simulink model "Furuta_Model"  (R2015a)
settings: Solver=ode3  SolverMode=SingleTasking  StartTime=0.0  StopTime=Inf  FixedStep=0.0001  RelTol=1e-3
PostLoadFcn:
  | , if any(exist('dsrtsu_mdlpostloadfcn', 'file') == [2, 3, 6]), try dsrtsu_mdlpostloadfcn('Execute', bdroot); catch fprintf('Error in PostLoadFcn (dsrtsu_mdlpostloadfcn) for model "%s":\n %s\n', bdroot, lasterr); end, end,
values from neighbouring files (symbols this model uses):
  alpha = J + (M+m1/3+m2)*L1^2    (= 0.002160093571)    [Furuta_Constants.m]
  beta = (M + m2/3)*L2^2    (= 0.00192796261667)    [Furuta_Constants.m]
  gamma = (M + m2/2)*L2*L1    (= 0.0009263333625)    [Furuta_Constants.m]
  initial_state = pi    (= 3.14159265359)    [Furuta_Constants.m]
  kb = 6e-4    (= 0.0006)    [Furuta_Constants.m]
  ke = 0.182    [Furuta_Constants.m]
  Re = 3.6    [Furuta_Constants.m]
  sigma = (M + m2/2)*g*L2    (= 0.0951054975)    [Furuta_Constants.m]
libraries: rti2202miolib x8, simulink_extras x1
settings Model: DSRTSU_INTERNAL_RTI_VER=450  DSRTSU_INTERNAL_RTI_TYPE=rti1006  DSRTSU_INTERNAL_RTIFPGA=40  CovMetricSettings=dwe  CovHtmlReporting=off  covSaveCumulativeToWorkspaceVar=off  CovSaveSingleToWorkspaceVar=off  CovExternalEMLEnable=on  Creator=Marcelo  LastModifiedBy=NSEE
settings SolverCC: ZeroCrossControl=DisableAll
settings DataIOCC: LimitDataPoints=off  SaveFormat=Dataset
settings OptimizationCC: BlockReduction=off  OptimizeBlockIOStorage=off  BufferReuse=off  GlobalBufferReuse=off  ExpressionFolding=off  LocalBlockOutputs=off
settings DebuggingCC: ParameterOverflowMsg=warning  SFUnexpectedBacktrackingDiag=error  SFNoUnconditionalDefaultTransitionDiag=error
settings HardwareCC: ProdBitPerPointer=64  ProdLargestAtomicFloat=Float  ProdIntDivRoundTo=Zero  ProdEndianess=LittleEndian  ProdHWDeviceType=Generic->Custom  TargetIntDivRoundTo=Zero  TargetEndianess=LittleEndian  TargetHWDeviceType=Generic->Custom
settings ModelReferenceCC: ModelReferenceMinAlgLoopOccurrences=on  PropagateSignalLabelsOutOfModel=on
settings RTWCC: SystemTargetFile=rti1006.tlc  MakeCommand=make_rti  TemplateMakefile=rti1006.tmf  Description=dSPACE DS1006 Hardware Platform
settings STFCustomTargetCC: GenerateSampleERTMain=off  ParMdlRefBuildCompliant=on  GeneratePreprocessorConditionals=Disable all  ERTCustomFileBanners=off  SupportNonInlinedSFcns=on  SupportVariableSizeSignals=off  MATLABClassNameForMDSCustomization=Simulink.SoftwareTarget.GRTCustomization  GRTInterface=on  SystemTargetFile=rti1006.tlc
settings GRTTargetCC: CompOptLevelCompliant=off  ConcurrentExecutionCompliant=off  CombineOutputUpdateFcns=off  MatFileLogging=off  CPPClassGenCompliant=off  GRTInterface=on  ExtModeMexFile=noextcomm

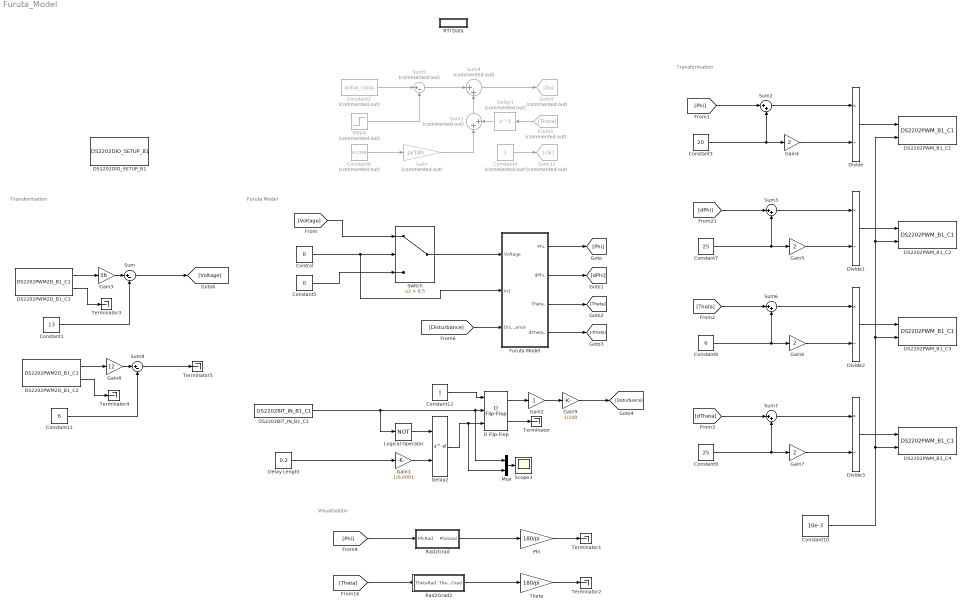
== system Furuta_Model ==
  note: Transformation
  note: Transformation
  note: Furuta Model
  note: Visualisation
  Constant1 : Constant  Value=13
  Constant10 : Constant  Value=10e-3
  Constant11 : Constant  Value=6
  Constant12 : Constant  OutDataTypeStr=boolean
  Constant2 : Constant  Commented=on  Value=initial_state
  Constant3 : Constant  Value=20
  Constant4 : Constant  Commented=on
  Constant5 : Constant  Value=0
  Constant6 : Constant  Commented=on  Value=9.2399
  Constant7 : Constant  Value=25
  Constant8 : Constant  Value=6
  Constant9 : Constant  Value=25
  Control : Constant  Value=0
  D Flip-Flop : simulink_extras/Flip Flops/D Flip-Flop
  DS2202BIT_IN_B1_C1 : rti2202miolib/DS2202BIT_IN_B1_C1  Reserved1=[]  Reserved2=[]  Reserved3=[]  Reserved4=[]  DSProperties=struct('RTI',struct('Version',uint32(1),'BlockType',struct('isSLSource',uint8(1),'isSLSink',uint8(0),'isHWSource',uint8(1),'isHWSink',uint8(0),'isSetup',uint8(0),'isInline',uint8(1),'isNonInline',uint8(0),'isInterrupt',uint8(0),'isChannelwise',uint8(1)),'IOBoardType',{{'DS2202','MIO'}},'UnitType','BIT','Identifier','BITINCH','DialogType','ML','BlockSet','NONE','SlaveProcessor','NONE'))  RTIBlockInterface=struct('OutputPortsWidth',int32(1),'OutputPortsDataType',{{'SS_BOOLEAN'}},'OutputPortsActive',1,'OutputPortsName',{{'BITCH_out'}},'BlockDisplay',{{['BIT IN\n Channelwise'],'center'}},'IconTransparency','off','InitLevel',2,'DialogFcn','gui2202bitinch','BlockName',struct('Token',{{'DS2202BIT_IN_B','_C'}},'BlockParam',{{'BoardNo','ChannelNo'}}),'MaskDescription',['Provides channelwise read access to the digital input.'])  RTIBlockParameters=struct('BoardNo',{{1,'ON',[1 16]}},'ChannelNo',{{1,'ON',[1 38]}},'TLCFileName',{{'rti2202inch','OFF',[]}})  RTISFcnParameters=struct('BoardNo','int32','ChannelNo','int32','TLCFileName','char')  RTIBlockParaDefault=struct('BoardNo',1,'ChannelNo',1,'TLCFileName','rti2202inch')
  DS2202DIO_SETUP_B1 : rti2202miolib/DS2202DIO_SETUP_B1  Reserved1=[]  Reserved2=[]  Reserved3=[]  Reserved4=[]  DSProperties=struct('RTI',struct('Version',uint32(2),'BlockType',struct('isSLSource',uint8(0),'isSLSink',uint8(0),'isHWSource',uint8(0),'isHWSink',uint8(0),'isSetup',uint8(1),'isInline',uint8(1),'isNonInline',uint8(0),'isInterrupt',uint8(0),'isChannelwise',uint8(0)),'IOBoardType',{{'DS2202','MIO'}},'UnitType','SETUP','Identifier','SETUP','DialogType','ML','BlockSet','NONE','SlaveProcessor','NONE'))  RTIBlockInterface=struct('OutputPortsWidth',int32(0),'OutputPortsActive',0,'BlockDisplay',{{['Digital I/O\n SETUP'],'center'}},'IconTransparency','on','InitLevel',2,'DialogFcn','gui2202diosetup','BlockName',struct('Token',{{'DS2202DIO_SETUP_B'}},'BlockParam',{{'BoardNo'}}),'MaskDescription',['Configures the threshold level and the termination mode for all digital IO'])  RTIBlockParameters=struct('BoardNo',{{1,'ON',[1 16]}},'TermMode',{{0,'OFF',[0 1]}},'BitInThresholdLevelCh1',{{'2.5','OFF',[1 23.8]}},'BitInThresholdLevelCh2',{{'2.5','OFF',[1 23.8]}},'BitInThresholdLevelCh3',{{'2.5','OFF',[1 23.8]}},'BitInThresholdLevelCh4',{{'2.5','OFF',[1 23.8]}},'BitInThresholdLevelCh5',{{'2.5','OFF',[1 23.8]}},'BitInThresholdLevelCh6',{{'2.5','OFF',[1 23.8]}},'BitInThresholdLevelCh7',{{'2.5','OFF',[1 23.8]}},'BitInThresholdLevelCh8',{{'2.5','OFF',[1 23.8]}},'BitInThresholdLevelCh9',{{'2.5','OFF',[1 23.8]}},'BitInThresholdLevelCh10',{{'2.5','OFF',[1 23.8]}},'BitInThresholdLevelCh11',{{'2.5','OFF',[1 23.8]}},'BitInThresholdLevelCh12',{{'2.5','OFF',[1 23.8]}},'BitInThresholdLevelCh13',{{'2.5','OFF',[1 23.8]}},'BitInThresholdLevelCh14',{{'2.5','OFF',[1 23.8]}},'BitInThresholdLevelCh15',{{'2.5','OFF',[1 23.8]}},'BitInThresholdLevelCh16',{{'2.5','OFF',[1 23.8]}},'BitInThresholdLevelCh17',{{'2.5','OFF',[1 23.8]}},'BitInThresholdLevelCh18',{{'2.5','OFF',[1 23.8]}},'BitInThresholdLevelCh19',{{'2.5','OFF',[1 23.8]}},'BitInThresholdLevelCh20',{{'2.5','OFF',[1 23.8]}},'BitInThresholdLevelCh21',{{'2.5','OFF',[1 23.8]}},'BitInThresholdLevelCh22',{{'2.5','OFF',[1 23.8]}},'BitInThresholdLevelCh23',{{'2.5','OFF',[1 23.8]}},'BitInThresholdLevelCh24',{{'2.5','OFF',[1 23.8]}},'BitInThresholdLevelCh25',{{'2.5','OFF',[1 23.8]}},'BitInThresholdLevelCh25_32',{{'2.5','OFF',[1 23.8]}},'BitInThresholdLevelCh33_38',{{'2.5','OFF',[1 23.8]}},'BitOutVBATRailsLOW',{{[1 1 1 1 1 1 1 1 1 1 1 1 1 1 1 1 1],'OFF',[]}},'BitOutVBATRailsVBAT1',{{[1 1 1 1 1 1 1 1 1 1 1 1 1 1 1 1 1],'OFF',[]}},'BitOutVBATRailsVBAT2',{{[0 0 0 0 0 0 0 0 0 0 0 0 0 0 0 0 0],'OFF',[]}},'PWMOutVBATRailsLOW',{{[1 1 1 1 1 1 1 1 1 1],'OFF',[]}},'PWMOutVBATRailsVBAT1',{{[1 1 1 1 1 1 1 1 1 1],'OFF',[]}},'PWMOutVBATRailsVBAT2',{{[0 0 0 0 0 0 0 0 0 0],'OFF',[]}},'TLCFileName',{{'rti2202setup','OFF',[]}})  RTISFcnParameters=struct('BoardNo','int32','TermMode','int32','BitInThresholdLevelCh1','double','BitInThresholdLevelCh2','double','BitInThresholdLevelCh3','double','BitInThresholdLevelCh4','double','BitInThresholdLevelCh5','double','BitInThresholdLevelCh6','double','BitInThresholdLevelCh7','double','BitInThresholdLevelCh8','double','BitInThresholdLevelCh9','double','BitInThresholdLevelCh10','double','BitInThresholdLevelCh11','double','BitInThresholdLevelCh12','double','BitInThresholdLevelCh13','double','BitInThresholdLevelCh14','double','BitInThresholdLevelCh15','double','BitInThresholdLevelCh16','double','BitInThresholdLevelCh17','double','BitInThresholdLevelCh18','double','BitInThresholdLevelCh19','double','BitInThresholdLevelCh20','double','BitInThresholdLevelCh21','double','BitInThresholdLevelCh22','double','BitInThresholdLevelCh23','double','BitInThresholdLevelCh24','double','BitInThresholdLevelCh25_32','double','BitInThresholdLevelCh33_38','double','BitOutVBATRailsLOW','int32','BitOutVBATRailsVBAT1','int32','BitOutVBATRailsVBAT2','int32','PWMOutVBATRailsLOW','int32','PWMOutVBATRailsVBAT1','int32','PWMOutVBATRailsVBAT2','int32','TLCFileName','char')  RTIBlockParaDefault=struct('BoardNo',1,'TermMode',0,'BitInThresholdLevelCh1',2.5,'BitInThresholdLevelCh2',2.5,'BitInThresholdLevelCh3',2.5,'BitInThresholdLevelCh4',2.5,'BitInThresholdLevelCh5',2.5,'BitInThresholdLevelCh6',2.5,'BitInThresholdLevelCh7',2.5,'BitInThresholdLevelCh8',2.5,'BitInThresholdLevelCh9',2.5,'BitInThresholdLevelCh10',2.5,'BitInThresholdLevelCh11',2.5,'BitInThresholdLevelCh12',2.5,'BitInThresholdLevelCh13',2.5,'BitInThresholdLevelCh14',2.5,'BitInThresholdLevelCh15',2.5,'BitInThresholdLevelCh16',2.5,'BitInThresholdLevelCh17',2.5,'BitInThresholdLevelCh18',2.5,'BitInThresholdLevelCh19',2.5,'BitInThresholdLevelCh20',2.5,'BitInThresholdLevelCh21',2.5,'BitInThresholdLevelCh22',2.5,'BitInThresholdLevelCh23',2.5,'BitInThresholdLevelCh24',2.5,'BitInThresholdLevelCh25',2.5,'BitInThresholdLevelCh25_32',2.5,'BitInThresholdLevelCh33_38',2.5,'BitOutVBATRailsLOW',[1 1 1 1 1 1 1 1 1 1 1 1 1 1 1 1 1],'BitOutVBATRailsVBAT1',[1 1 1 1 1 1 1 1 1 1 1 1 1 1 1 1 1],'BitOutVBATRailsVBAT2',[0 0 0 0 0 0 0 0 0 0 0 0 0 0 0 0 0],'PWMOutVBATRailsLOW',[1 1 1 1 1 1 1 1 1 1],'PWMOutVBATRailsVBAT1',[1 1 1 1 1 1 1 1 1 1],'PWMOutVBATRailsVBAT2',[0 0 0 0 0 0 0 0 0 0],'TLCFileName','rti2202setup')
  DS2202PWM2D_B1_C1 : rti2202miolib/DS2202PWM2D_B1_C1  Reserved1=[]  Reserved2=[]  Reserved3=[]  Reserved4=[]  DSProperties=struct('RTI',struct('Version',uint32(1),'BlockType',struct('isSLSource',uint8(1),'isSLSink',uint8(0),'isHWSource',uint8(1),'isHWSink',uint8(0),'isSetup',uint8(0),'isInline',uint8(1),'isNonInline',uint8(0),'isInterrupt',uint8(0),'isChannelwise',uint8(1)),'IOBoardType',{{'DS2202','MIO'}},'UnitType','PWM','Identifier','PWM2D','DialogType','ML','BlockSet','NONE','SlaveProcessor','NONE'))  RTIBlockInterface=struct('OutputPortsWidth',int32([1 1]),'OutputPortsActive',[1 1],'OutputPortsName',{{['Duty Cycle'],'Period'}},'IconTransparency','on','InitLevel',2,'DialogFcn','gui2202pwm2d','BlockName',struct('Token',{{'DS2202PWM2D_B','_C'}},'BlockParam',{{'BoardNo','ChannelNo'}}),'MaskDescription',['Provides read access to the pulse width of square-wave-type signals.'])  RTIBlockParameters=struct('BoardNo',{{1,'ON',[1 16]}},'ChannelNo',{{1,'ON',[1 24]}},'UpdateMode',{{1,'ON',[1 2]}},'PeriodRange',{{3,'OFF',[1 16]}},'TLCFileName',{{'rti2202pwm2d','OFF',[]}})  RTISFcnParameters=struct('BoardNo','int32','ChannelNo','int32','UpdateMode','int32','PeriodRange','int32','TLCFileName','char')  RTIBlockParaDefault=struct('BoardNo',1,'ChannelNo',1,'UpdateMode',1,'PeriodRange',7,'TLCFileName','rti2202pwm2d')
  DS2202PWM2D_B1_C2 : rti2202miolib/DS2202PWM2D_B1_C1  Reserved1=[]  Reserved2=[]  Reserved3=[]  Reserved4=[]  DSProperties=struct('RTI',struct('Version',uint32(1),'BlockType',struct('isSLSource',uint8(1),'isSLSink',uint8(0),'isHWSource',uint8(1),'isHWSink',uint8(0),'isSetup',uint8(0),'isInline',uint8(1),'isNonInline',uint8(0),'isInterrupt',uint8(0),'isChannelwise',uint8(1)),'IOBoardType',{{'DS2202','MIO'}},'UnitType','PWM','Identifier','PWM2D','DialogType','ML','BlockSet','NONE','SlaveProcessor','NONE'))  RTIBlockInterface=struct('OutputPortsWidth',int32([1 1]),'OutputPortsActive',[1 1],'OutputPortsName',{{['Duty Cycle'],'Period'}},'IconTransparency','on','InitLevel',2,'DialogFcn','gui2202pwm2d','BlockName',struct('Token',{{'DS2202PWM2D_B','_C'}},'BlockParam',{{'BoardNo','ChannelNo'}}),'MaskDescription',['Provides read access to the pulse width of square-wave-type signals.'])  RTIBlockParameters=struct('BoardNo',{{1,'ON',[1 16]}},'ChannelNo',{{2,'ON',[1 24]}},'UpdateMode',{{1,'ON',[1 2]}},'PeriodRange',{{3,'OFF',[1 16]}},'TLCFileName',{{'rti2202pwm2d','OFF',[]}})  RTISFcnParameters=struct('BoardNo','int32','ChannelNo','int32','UpdateMode','int32','PeriodRange','int32','TLCFileName','char')  RTIBlockParaDefault=struct('BoardNo',1,'ChannelNo',1,'UpdateMode',1,'PeriodRange',7,'TLCFileName','rti2202pwm2d')
  DS2202PWM_B1_C1 : rti2202miolib/DS2202PWM_B1_C1  Reserved1=[]  Reserved2=[]  Reserved3=[]  Reserved4=[]  DSProperties=struct('RTI',struct('Version',uint32(1),'BlockType',struct('isSLSource',uint8(0),'isSLSink',uint8(1),'isHWSource',uint8(0),'isHWSink',uint8(1),'isSetup',uint8(0),'isInline',uint8(1),'isNonInline',uint8(0),'isInterrupt',uint8(0),'isChannelwise',uint8(1)),'IOBoardType',{{'DS2202','MIO'}},'UnitType','PWM','Identifier','PWM','DialogType','ML','BlockSet','NONE','SlaveProcessor','NONE'))  RTIBlockInterface=struct('InputPortsWidth',int32([1 1]),'InputPortsActive',[1 1],'InputPortsName',{{['Duty Cycle'],'Period'}},'IconTransparency','on','InitLevel',2,'DialogFcn','gui2202pwm','BlockName',struct('Token',{{'DS2202PWM_B','_C'}},'BlockParam',{{'BoardNo','ChannelNo'}}),'MaskDescription',['Generation of a square-wave-type signal for a given period and duty cycle.'])  RTIBlockParameters=struct('BoardNo',{{1,'ON',[1 16]}},'ChannelNo',{{1,'ON',[1 9]}},'UpdateMode',{{1,'ON',[1 2]}},'PeriodRange',{{3,'OFF',[1 16]}},'DutyCycleInitValue',{{'0','OFF',[0 1]}},'PeriodInitValue',{{'5e-05','OFF',[]}},'DutyCyclePeriodTermMode',{{0,'OFF',[0 1]}},'DutyCycleTermValue',{{'0','OFF',[0 1]}},'PeriodTermValue',{{'5e-05','OFF',[]}},'TLCFileName',{{'rti2202pwm','OFF',[]}})  RTISFcnParameters=struct('BoardNo','int32','ChannelNo','int32','UpdateMode','int32','PeriodRange','int32','DutyCycleInitValue','double','PeriodInitValue','double','DutyCyclePeriodTermMode','int32','DutyCycleTermValue','double','PeriodTermValue','double','TLCFileName','char')  RTIBlockParaDefault=struct('BoardNo',1,'ChannelNo',1,'UpdateMode',1,'PeriodRange',7,'DutyCycleInitValue',0,'PeriodInitValue',5e-05,'DutyCyclePeriodTermMode',0,'DutyCycleTermValue',0,'PeriodTermValue',5e-05,'TLCFileName','rti2202pwm')
  DS2202PWM_B1_C2 : rti2202miolib/DS2202PWM_B1_C1  Reserved1=[]  Reserved2=[]  Reserved3=[]  Reserved4=[]  DSProperties=struct('RTI',struct('Version',uint32(1),'BlockType',struct('isSLSource',uint8(0),'isSLSink',uint8(1),'isHWSource',uint8(0),'isHWSink',uint8(1),'isSetup',uint8(0),'isInline',uint8(1),'isNonInline',uint8(0),'isInterrupt',uint8(0),'isChannelwise',uint8(1)),'IOBoardType',{{'DS2202','MIO'}},'UnitType','PWM','Identifier','PWM','DialogType','ML','BlockSet','NONE','SlaveProcessor','NONE'))  RTIBlockInterface=struct('InputPortsWidth',int32([1 1]),'InputPortsActive',[1 1],'InputPortsName',{{['Duty Cycle'],'Period'}},'IconTransparency','on','InitLevel',2,'DialogFcn','gui2202pwm','BlockName',struct('Token',{{'DS2202PWM_B','_C'}},'BlockParam',{{'BoardNo','ChannelNo'}}),'MaskDescription',['Generation of a square-wave-type signal for a given period and duty cycle.'])  RTIBlockParameters=struct('BoardNo',{{1,'ON',[1 16]}},'ChannelNo',{{2,'ON',[1 9]}},'UpdateMode',{{1,'ON',[1 2]}},'PeriodRange',{{3,'OFF',[1 16]}},'DutyCycleInitValue',{{'0','OFF',[0 1]}},'PeriodInitValue',{{'5e-05','OFF',[]}},'DutyCyclePeriodTermMode',{{0,'OFF',[0 1]}},'DutyCycleTermValue',{{'0','OFF',[0 1]}},'PeriodTermValue',{{'5e-05','OFF',[]}},'TLCFileName',{{'rti2202pwm','OFF',[]}})  RTISFcnParameters=struct('BoardNo','int32','ChannelNo','int32','UpdateMode','int32','PeriodRange','int32','DutyCycleInitValue','double','PeriodInitValue','double','DutyCyclePeriodTermMode','int32','DutyCycleTermValue','double','PeriodTermValue','double','TLCFileName','char')  RTIBlockParaDefault=struct('BoardNo',1,'ChannelNo',1,'UpdateMode',1,'PeriodRange',7,'DutyCycleInitValue',0,'PeriodInitValue',5e-05,'DutyCyclePeriodTermMode',0,'DutyCycleTermValue',0,'PeriodTermValue',5e-05,'TLCFileName','rti2202pwm')
  DS2202PWM_B1_C3 : rti2202miolib/DS2202PWM_B1_C1  Reserved1=[]  Reserved2=[]  Reserved3=[]  Reserved4=[]  DSProperties=struct('RTI',struct('Version',uint32(1),'BlockType',struct('isSLSource',uint8(0),'isSLSink',uint8(1),'isHWSource',uint8(0),'isHWSink',uint8(1),'isSetup',uint8(0),'isInline',uint8(1),'isNonInline',uint8(0),'isInterrupt',uint8(0),'isChannelwise',uint8(1)),'IOBoardType',{{'DS2202','MIO'}},'UnitType','PWM','Identifier','PWM','DialogType','ML','BlockSet','NONE','SlaveProcessor','NONE'))  RTIBlockInterface=struct('InputPortsWidth',int32([1 1]),'InputPortsActive',[1 1],'InputPortsName',{{['Duty Cycle'],'Period'}},'IconTransparency','on','InitLevel',2,'DialogFcn','gui2202pwm','BlockName',struct('Token',{{'DS2202PWM_B','_C'}},'BlockParam',{{'BoardNo','ChannelNo'}}),'MaskDescription',['Generation of a square-wave-type signal for a given period and duty cycle.'])  RTIBlockParameters=struct('BoardNo',{{1,'ON',[1 16]}},'ChannelNo',{{3,'ON',[1 9]}},'UpdateMode',{{1,'ON',[1 2]}},'PeriodRange',{{3,'OFF',[1 16]}},'DutyCycleInitValue',{{'0','OFF',[0 1]}},'PeriodInitValue',{{'5e-05','OFF',[]}},'DutyCyclePeriodTermMode',{{0,'OFF',[0 1]}},'DutyCycleTermValue',{{'0','OFF',[0 1]}},'PeriodTermValue',{{'5e-05','OFF',[]}},'TLCFileName',{{'rti2202pwm','OFF',[]}})  RTISFcnParameters=struct('BoardNo','int32','ChannelNo','int32','UpdateMode','int32','PeriodRange','int32','DutyCycleInitValue','double','PeriodInitValue','double','DutyCyclePeriodTermMode','int32','DutyCycleTermValue','double','PeriodTermValue','double','TLCFileName','char')  RTIBlockParaDefault=struct('BoardNo',1,'ChannelNo',1,'UpdateMode',1,'PeriodRange',7,'DutyCycleInitValue',0,'PeriodInitValue',5e-05,'DutyCyclePeriodTermMode',0,'DutyCycleTermValue',0,'PeriodTermValue',5e-05,'TLCFileName','rti2202pwm')
  DS2202PWM_B1_C4 : rti2202miolib/DS2202PWM_B1_C1  Reserved1=[]  Reserved2=[]  Reserved3=[]  Reserved4=[]  DSProperties=struct('RTI',struct('Version',uint32(1),'BlockType',struct('isSLSource',uint8(0),'isSLSink',uint8(1),'isHWSource',uint8(0),'isHWSink',uint8(1),'isSetup',uint8(0),'isInline',uint8(1),'isNonInline',uint8(0),'isInterrupt',uint8(0),'isChannelwise',uint8(1)),'IOBoardType',{{'DS2202','MIO'}},'UnitType','PWM','Identifier','PWM','DialogType','ML','BlockSet','NONE','SlaveProcessor','NONE'))  RTIBlockInterface=struct('InputPortsWidth',int32([1 1]),'InputPortsActive',[1 1],'InputPortsName',{{['Duty Cycle'],'Period'}},'IconTransparency','on','InitLevel',2,'DialogFcn','gui2202pwm','BlockName',struct('Token',{{'DS2202PWM_B','_C'}},'BlockParam',{{'BoardNo','ChannelNo'}}),'MaskDescription',['Generation of a square-wave-type signal for a given period and duty cycle.'])  RTIBlockParameters=struct('BoardNo',{{1,'ON',[1 16]}},'ChannelNo',{{4,'ON',[1 9]}},'UpdateMode',{{1,'ON',[1 2]}},'PeriodRange',{{3,'OFF',[1 16]}},'DutyCycleInitValue',{{'0','OFF',[0 1]}},'PeriodInitValue',{{'5e-05','OFF',[]}},'DutyCyclePeriodTermMode',{{0,'OFF',[0 1]}},'DutyCycleTermValue',{{'0','OFF',[0 1]}},'PeriodTermValue',{{'5e-05','OFF',[]}},'TLCFileName',{{'rti2202pwm','OFF',[]}})  RTISFcnParameters=struct('BoardNo','int32','ChannelNo','int32','UpdateMode','int32','PeriodRange','int32','DutyCycleInitValue','double','PeriodInitValue','double','DutyCyclePeriodTermMode','int32','DutyCycleTermValue','double','PeriodTermValue','double','TLCFileName','char')  RTIBlockParaDefault=struct('BoardNo',1,'ChannelNo',1,'UpdateMode',1,'PeriodRange',7,'DutyCycleInitValue',0,'PeriodInitValue',5e-05,'DutyCyclePeriodTermMode',0,'DutyCycleTermValue',0,'PeriodTermValue',5e-05,'TLCFileName','rti2202pwm')
  Delay Lenght : Constant  Value=0.2  OutDataTypeStr=double
  Delay1 : Delay  Commented=on  DelayLength=1
  Delay2 : Delay  DelayLengthSource=Input port  DelayLengthUpperLimit=100000  InitialCondition=1
      settings: InputPortMap=u0,p1
  Divide{,1..3} (4 alike) : Product  Inputs=*/
  From5 : From  Commented=on  GotoTag=Theta
  "Furuta Model " : Subsystem
  Gain : Gain  Commented=on  Gain=pi/180
  Gain1 : Gain  Gain=1/0.0001
  Gain2 : Gain  ParamDataTypeStr=double
  Gain3 : Gain  Gain=26
  Gain{4..7} (4 alike) : Gain  Gain=2
  Gain8 : Gain  Gain=12
  Gain9 : Gain  Gain=1/100
  Goto11 : Goto  Commented=on  GotoTag=clk
  Goto5 : Goto  Commented=on  GotoTag=Xo
  Logical Operator : Logic  Operator=NOT  AllPortsSameDT=off  OutDataTypeStr=boolean
  Mux : Mux  Inputs=2
  Phi : Gain  Gain=180/pi
  RTI Data : Subsystem  Tag=struct('RTIDataServer',struct('RTIDataServerVs','2','RTIModelDescription','struct(''main'',''Furuta_Model'',''sub'','''',''isMp'',0)'))  LoadFcn="if exist('rtidc'), try,  rtidc('DataHostBlockClbLoad', gcbh); catch, disp(['Warning: ''LoadFcn'' for RTI Data block failed: ' lasterr]); end, end,"  mask(RTI_DATA_HOST){}
      mask help:
      | RTI Data Block.
      | This block is used by RTI to store internal model-dependent data.
      | Please keep this block on the root level of the model. Deleting this block will result in data loss.
      |
      | NEVER DELETE OR COPY THIS BLOCK!
      settings: CopyFcn="if exist('rtidc'), try,  rtidc('DataHostBlockClbCopy', gcbh); catch, disp(['Warning: ''CopyFcn'' for RTI Data block failed: ' lasterr]); end, end,"  DeleteFcn="if exist('rtidc'), try,  rtidc('DataHostBlockClbDelete', gcbh); catch, disp(['Warning: ''DeleteFcn'' for RTI Data block failed: ' lasterr]); end, end,"  ModelCloseFcn="if exist('rtidc'), try,  rtidc('DataHostBlockClbModelClose', gcbh); catch, disp(['Warning: ''ModelCloseFcn'' for RTI Data block failed: ' lasterr]); end, end,"  PreSaveFcn="if exist('rtidc'), try,  rtidc('DataHostBlockClbPreSave', gcbh); catch, disp(['Warning: ''PreSaveFcn'' for RTI Data block failed: ' lasterr]); end, end,"  PostSaveFcn="if exist('rtidc'), try,  rtidc('DataHostBlockClbPostSave', gcbh); catch, disp(['Warning: ''PostSaveFcn'' for RTI Data block failed: ' lasterr]); end, end,"  NameChangeFcn="if exist('rtidc'), try,  rtidc('DataHostBlockClbNameChange', gcbh); catch, disp(['Warning: ''NameChangeFcn'' for RTI Data block failed: ' lasterr]); end, end,"
      mask Help:
      | RTI Data Block.
      | This block is used by RTI to store internal model-dependent data.
      | Please keep this block on the root level of the model. Deleting this block will result in data loss.
      | 
      | NEVER DELETE OR COPY THIS BLOCK!
      mask Display:
      | text(0.5, 0.5, 'RTI Data', 'HorizontalAlignment', 'center');
      | plot([1 0]);
  Rad2Grad : Subsystem
  Rad2Grad2 : Subsystem
  Scope3 : Scope
      settings: TimeRange=10  SaveName=ScopeData3
  Step4 : Step  Commented=on  Time=0.5  After=initial_state  SampleTime=0
  Sum : Sum  Inputs=|+-
  Sum1 : Sum  Commented=on  Inputs=|++
  Sum{2..3,6..7} (4 alike) : Sum  Inputs=|++
  Sum4 : Sum  Commented=on  Inputs=|++
  Sum5 : Sum  Commented=on  Inputs=|+-
  Sum8 : Sum  Inputs=|+-
  Switch : Switch  Criteria=u2 > Threshold  Threshold=0.5
  Terminator{,1..5} (6 alike) : Terminator
  Theta : Gain  Gain=180/pi
  wires:
  "Furuta Model "/1(Phi.) -> [Phi]
  "Furuta Model "/2(dPhi.) -> [dPhi]
  "Furuta Model "/3(Theta.) -> [Theta]
  [Phi] -> Rad2Grad/1(PhiRad)
  [Theta] -> Rad2Grad2/1(ThetaRad)
  Rad2Grad2/1(ThetaGrad) -> Theta/1
  Rad2Grad/1(PhiGrad) -> Phi/1
  "Furuta Model "/4(dTheta.) -> [dTheta]
  Step4/1 -> Sum5/2
  Sum4/1 -> Goto5/1
  Sum5/1 -> Sum4/1
  Constant2/1 -> Sum5/1
  Constant6/1 -> Gain/1
  [Voltage] -> Switch/1
  Switch/1 -> "Furuta Model "/1("Voltage ")
  Control/1 -> "Furuta Model "/2(In1), Switch/2
  Constant5/1 -> Switch/3
  Constant4/1 -> Goto11/1
  From5/1 -> Delay1/1
  Gain/1 -> Sum1/1
  Sum1/1 -> Sum4/2
  Delay1/1 -> Sum1/2
  Theta/1 -> Terminator2/1
  Phi/1 -> Terminator1/1
  DS2202PWM2D_B1_C1/1 -> Gain3/1
  Gain3/1 -> Sum/1
  Constant1/1 -> Sum/2
  [Phi] -> Sum2/1
  Sum2/1 -> Divide/1
  Constant3/1 -> Gain4/1, Sum2/2
  Gain4/1 -> Divide/2
  [dPhi] -> Sum3/1
  Sum3/1 -> Divide1/1
  Constant7/1 -> Gain5/1, Sum3/2
  Gain5/1 -> Divide1/2
  [Theta] -> Sum6/1
  Sum6/1 -> Divide2/1
  Constant8/1 -> Gain6/1, Sum6/2
  Gain6/1 -> Divide2/2
  [dTheta] -> Sum7/1
  Sum7/1 -> Divide3/1
  Constant9/1 -> Gain7/1, Sum7/2
  Gain7/1 -> Divide3/2
  Divide2/1 -> DS2202PWM_B1_C3/1
  Divide3/1 -> DS2202PWM_B1_C4/1
  Divide/1 -> DS2202PWM_B1_C1/1
  Divide1/1 -> DS2202PWM_B1_C2/1
  Constant10/1 -> DS2202PWM_B1_C4/2, DS2202PWM_B1_C3/2, DS2202PWM_B1_C2/2, DS2202PWM_B1_C1/2
  DS2202PWM2D_B1_C1/2 -> Terminator3/1
  Sum/1 -> [Voltage]
  DS2202PWM2D_B1_C2/1 -> Gain8/1
  Gain8/1 -> Sum8/1
  Constant11/1 -> Sum8/2
  DS2202PWM2D_B1_C2/2 -> Terminator4/1
  Sum8/1 -> Terminator5/1
  Constant12/1 -> D Flip-Flop/1
  Delay2/1 -> Mux/2, D Flip-Flop/3
  Logical Operator/1 -> Delay2/1
  D Flip-Flop/1 -> Gain2/1
  Gain2/1 -> Gain9/1
  D Flip-Flop/2 -> Terminator/1
  Delay Lenght/1 -> Gain1/1
  Mux/1 -> Scope3/1
  Gain1/1 -> Delay2/2
  Gain9/1 -> [Disturbance]
  [Disturbance] -> "Furuta Model "/3(Disturbance)
  DS2202BIT_IN_B1_C1/1 -> Logical Operator/1, Mux/1, D Flip-Flop/2

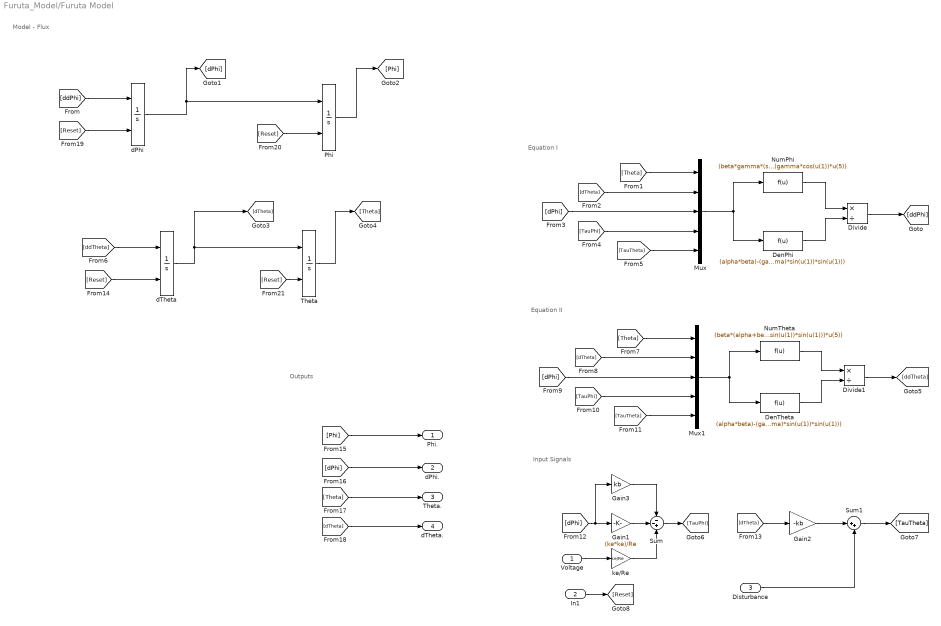
== system Furuta_Model/Furuta Model  ==
  note: Outputs
  note: Input Signals
  note: Equation II
  note: Equation I
  note: Model - Flux
  "Voltage " : Inport
  In1 : Inport  Port=2
  Disturbance : Inport  Port=3
  DenPhi : Fcn  Expr=(alpha*beta)-(gamma*gamma)+((beta*beta+gamma*gamma)*sin(u(1))*sin(u(1)))
  DenTheta : Fcn  Expr=(alpha*beta)-(gamma*gamma)+((beta*beta+gamma*gamma)*sin(u(1))*sin(u(1)))
  Divide : Product  Inputs=*/
  Divide1 : Product  Inputs=*/
  Gain1 : Gain  Gain=(ke*ke)/Re
  Gain2 : Gain  Gain=-kb
  Gain3 : Gain  Gain=kb
  Mux : Mux  Inputs=5
  Mux1 : Mux  Inputs=5
  NumPhi : Fcn  Expr=(beta*gamma*(sin(u(1))*sin(u(1))-1)*sin(u(1))*u(3)*u(3))-(2*beta*beta*cos(u(1))*sin(u(1))*u(3)*u(2))+(beta*gamma*sin(u(1))*u(2)*u(2))-(gamma*sigma*cos(u(1))*sin(u(1)))+(beta*u(4))-(gamma*cos(u(1))*u(5))
  NumTheta : Fcn  Expr=(beta*(alpha+beta*sin(u(1))*sin(u(1)))*cos(u(1))*sin(u(1))*u(3)*u(3))+(2*beta*gamma*(1-sin(u(1))*sin(u(1)))*sin(u(1))*u(3)*u(2))-(gamma*gamma*cos(u(1))*sin(u(1))*u(2)*u(2))+(sigma*(alpha+beta*sin(u(1))*sin(u(1)))*sin(u(1)))-(gamma*cos(u(1))*u(4))+((alpha+beta*sin(u(1))*sin(u(1)))*u(5))
  Phi : Integrator  ExternalReset=rising
  Sum : Sum  Inputs=--+
  Sum1 : Sum  Inputs=|++
  Theta : Integrator  ExternalReset=rising  InitialCondition=initial_state
  dPhi : Integrator  ExternalReset=rising
  dTheta : Integrator  ExternalReset=rising
  "ke/Re " : Gain  Gain=ke/Re
  Phi. : Outport
  dPhi. : Outport  Port=2
  Theta. : Outport  Port=3
  dTheta. : Outport  Port=4
  wires:
  Divide/1 -> [ddPhi]
  "ke/Re "/1 -> Sum/3
  Sum/1 -> [TauPhi]
  Gain1/1 -> Sum/2
  "Voltage "/1 -> "ke/Re "/1
  [dTheta] -> Gain2/1
  Gain3/1 -> Sum/1
  dTheta/1 -> [dTheta], Theta/1
  [Theta] -> Mux1/1
  Mux1/1 -> DenTheta/1, NumTheta/1
  [dTheta] -> Mux1/2
  [dPhi] -> Mux1/3
  [TauTheta] -> Mux1/5
  [TauPhi] -> Mux1/4
  [Theta] -> Mux/1
  [TauTheta] -> Mux/5
  [TauPhi] -> Mux/4
  Phi/1 -> [Phi]
  [dPhi] -> Mux/3
  DenPhi/1 -> Divide/2
  [ddPhi] -> dPhi/1
  [ddTheta] -> dTheta/1
  dPhi/1 -> Phi/1, [dPhi]
  NumTheta/1 -> Divide1/1
  NumPhi/1 -> Divide/1
  DenTheta/1 -> Divide1/2
  Mux/1 -> DenPhi/1, NumPhi/1
  [dPhi] -> Gain3/1, Gain1/1
  [dTheta] -> Mux/2
  Divide1/1 -> [ddTheta]
  [Phi] -> Phi./1
  [dPhi] -> dPhi./1
  [Theta] -> Theta./1
  [dTheta] -> dTheta./1
  In1/1 -> [Reset]
  [Reset] -> dTheta/2
  [Reset] -> dPhi/2
  [Reset] -> Phi/2
  [Reset] -> Theta/2
  Theta/1 -> [Theta]
  Gain2/1 -> Sum1/1
  Sum1/1 -> [TauTheta]
  Disturbance/1 -> Sum1/2

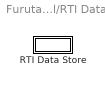
== system Furuta_Model/RTI Data ==
  RTI Data Store : Subsystem  Tag="struct('private',struct('version',struct('dsVer',uint32(2),'dsVerCreation',uint32(2),'RTI',struct('ver','7.3','type','RTI1006')),'access',struct('type','Model','isPerm',1,'created',['02-Oct-2018 16:40:55'],'modified',['06-Nov-2018 13:55:35'],'location','')),'public',struct('main',struct('data',[]),'sub',struct('name',{{'Furuta_Model'}},'data',{{struct('TH',struct('thTaskInfo',struct('taskType',{'TIMER','HWINT','TMRINT','SWINT','GLINT'},'tasksNumOf',{1,0,0,0,0},'srcIds',{{'TIMERA'},{},{},{},{}},'taskNames',{{['Timer Task 1']},{},{},{},{}})),'th_tc',struct('dataType','TASK','taskGroupId','','taskGroupList',{{}},'taskSchedulingPolicy','FCFS','taskType','TIMER','blkh',-1,'srcId','TIMERA','srcSgnName',['Timer A interrupt'],'srcCpuName','','taskName',['Timer Task 1  [0.0001] s'],'taskNameDisplayExt','','smplTime',0.0001,'smplTimeOffs',0,'hasFixedPriority',0,'priority',1,'hasFixedOvc',0,'ovcType',1,'ovcMax',1),'tc_th',struct('dataType','TASK','taskGroupId','','taskGroupList',{{}},'taskSchedulingPolicy','FCFS','taskType','TIMER','blkh',-1,'srcId','TIMERA','srcSgnName',['Timer A interrupt'],'srcCpuName','','taskName',['Timer Task 1  [0.0001] s'],'taskNameDisplayExt','','smplTime',0.0001,'smplTimeOffs',0,'hasFixedPriority',0,'priority',1,'hasFixedOvc',0,'ovcType',1,'ovcMax',1))}})))"  mask(RTI_DATA_STORE){}
      mask help:
      | RTI Data Store Block. This block is used by RTI to store internal model dependent data. Deleting this block will result in data loss.
      |
      | NEVER DELETE, COPY, OR MODIFY THIS BLOCK!
      mask Help:
      | RTI Data Store Block. This block is used by RTI to store internal model dependent data. Deleting this block will result in data loss.
      | 
      | NEVER DELETE, COPY, OR MODIFY THIS BLOCK!
      mask Display: text(0.5, 0.5, ' ', 'HorizontalAlignment', 'center');

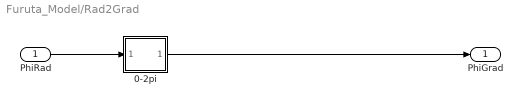
== system Furuta_Model/Rad2Grad ==
  PhiRad : Inport
  0-2pi : Subsystem
  PhiGrad : Outport
  wires:
  0-2pi/1(Out1) -> PhiGrad/1
  PhiRad/1 -> 0-2pi/1(In1)

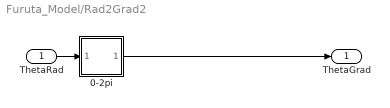
== system Furuta_Model/Rad2Grad2 ==
  ThetaRad : Inport
  0-2pi : Subsystem
  ThetaGrad : Outport
  wires:
  ThetaRad/1 -> 0-2pi/1(In1)
  0-2pi/1(Out1) -> ThetaGrad/1

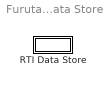
== system Furuta_Model/RTI Data/RTI Data Store ==
  RTI Data Store : Subsystem  mask(RTI_DATA_STORE){}
      mask help:
      | RTI Data Store Block. This block is used by RTI to store internal model dependent data. Deleting this block will result in data loss.
      |
      | NEVER DELETE, COPY, OR MODIFY THIS BLOCK!
      mask Help:
      | RTI Data Store Block. This block is used by RTI to store internal model dependent data. Deleting this block will result in data loss.
      | 
      | NEVER DELETE, COPY, OR MODIFY THIS BLOCK!
      mask Display: text(0.5, 0.5, ' ', 'HorizontalAlignment', 'center');

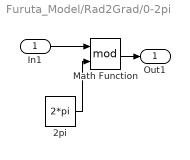
== system Furuta_Model/Rad2Grad/0-2pi ==
  In1 : Inport
  2pi : Constant  Value=2*pi
  Math Function : Math  Operator=mod  SaturateOnIntegerOverflow=on
  Out1 : Outport
  wires:
  2pi/1 -> Math Function/2
  Math Function/1 -> Out1/1
  In1/1 -> Math Function/1

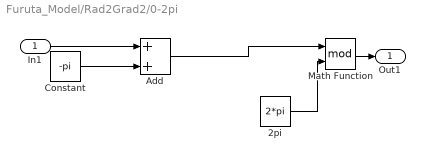
== system Furuta_Model/Rad2Grad2/0-2pi ==
  In1 : Inport
  2pi : Constant  Value=2*pi
  Add : Sum
  Constant : Constant  Value=-pi
  Math Function : Math  Operator=mod  SaturateOnIntegerOverflow=on
  Out1 : Outport
  wires:
  Math Function/1 -> Out1/1
  2pi/1 -> Math Function/2
  Constant/1 -> Add/2
  In1/1 -> Add/1
  Add/1 -> Math Function/1

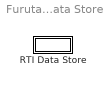
== system Furuta_Model/RTI Data/RTI Data Store/RTI Data Store ==
  RTI Data Store : Subsystem  mask(RTI_DATA_STORE){}
      mask help:
      | RTI Data Store Block. This block is used by RTI to store internal model dependent data. Deleting this block will result in data loss.
      |
      | NEVER DELETE, COPY, OR MODIFY THIS BLOCK!
      mask Help:
      | RTI Data Store Block. This block is used by RTI to store internal model dependent data. Deleting this block will result in data loss.
      | 
      | NEVER DELETE, COPY, OR MODIFY THIS BLOCK!
      mask Display: text(0.5, 0.5, ' ', 'HorizontalAlignment', 'center');

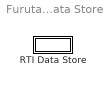
== system Furuta_Model/RTI Data/RTI Data Store/RTI Data Store/RTI Data Store ==
  RTI Data Store : Subsystem  mask(RTI_DATA_STORE){}
      mask help:
      | RTI Data Store Block. This block is used by RTI to store internal model dependent data. Deleting this block will result in data loss.
      |
      | NEVER DELETE, COPY, OR MODIFY THIS BLOCK!
      mask Help:
      | RTI Data Store Block. This block is used by RTI to store internal model dependent data. Deleting this block will result in data loss.
      | 
      | NEVER DELETE, COPY, OR MODIFY THIS BLOCK!
      mask Display: text(0.5, 0.5, ' ', 'HorizontalAlignment', 'center');

== system Furuta_Model/RTI Data/RTI Data Store/RTI Data Store/RTI Data Store/RTI Data Store ==
